simulink library "FoldingMechanisms"  (R2017a)
settings: Solver=VariableStepAuto  StartTime=0.0  StopTime=10.0  RelTol=1e-3
undefined symbols (not defined in the file or in its folder): X, Y, Z
libraries: sm_lib x70, FoldingMechanisms x62, nesl_utility x7
(part 4 of 4)

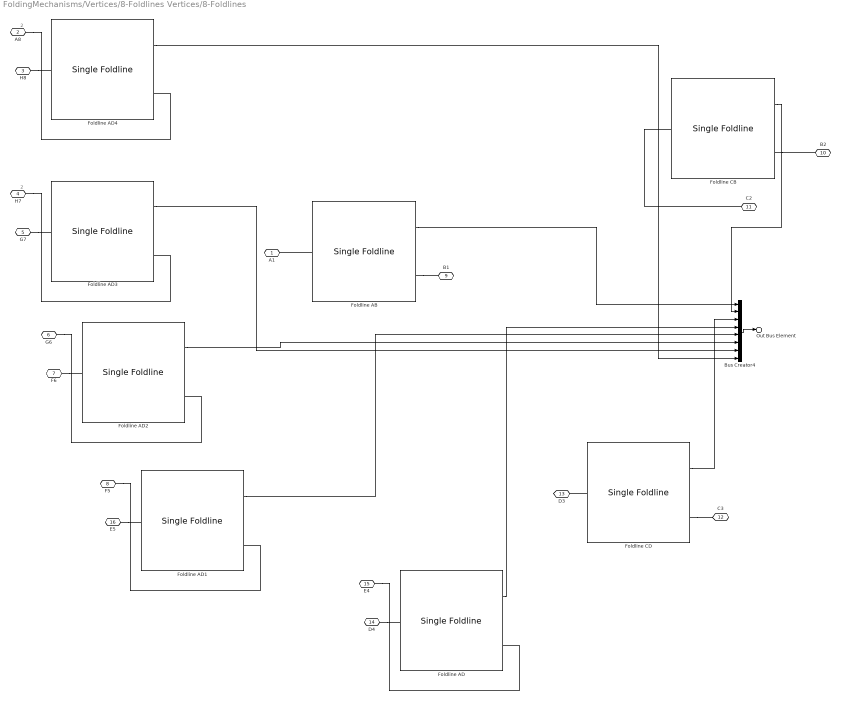
== system FoldingMechanisms/Vertices/8-Foldlines Vertices/8-Foldlines ==
  note: 2
  note: 2
  Bus Creator4 : BusCreator  Inputs=8
  Foldline AB : FoldingMechanisms/Vertices/Subelements/Single Foldline  angleAB=angval(1)  specAngleAB=angspec(1)
      settings: SourceProductName=FoldingMechanisms
  Foldline AD{,1..4} (5 alike) : FoldingMechanisms/Vertices/Subelements/Single Foldline  angleAB=angval(4)  specAngleAB=angspec(4)
      settings: SourceProductName=FoldingMechanisms
  Foldline CB : FoldingMechanisms/Vertices/Subelements/Single Foldline  angleAB=angval(2)  specAngleAB=angspec(2)
      settings: SourceProductName=FoldingMechanisms
  Foldline CD : FoldingMechanisms/Vertices/Subelements/Single Foldline  angleAB=angval(3)  specAngleAB=angspec(2)
      settings: SourceProductName=FoldingMechanisms
  A1 : PMIOPort  Port=1  Side=Left
  A8 : PMIOPort  Port=2  Side=Left
  H8 : PMIOPort  Port=3  Side=Left
  H7 : PMIOPort  Port=4  Side=Left
  G7 : PMIOPort  Port=5  Side=Left
  G6 : PMIOPort  Port=6  Side=Left
  F6 : PMIOPort  Port=7  Side=Left
  F5 : PMIOPort  Port=8  Side=Left
  B1 : PMIOPort  Port=9  Side=Right
  B2 : PMIOPort  Port=10  Side=Right
  C2 : PMIOPort  Port=11  Side=Right
  C3 : PMIOPort  Port=12  Side=Right
  D3 : PMIOPort  Port=13  Side=Right
  D4 : PMIOPort  Port=14  Side=Right
  E4 : PMIOPort  Port=15  Side=Right
  E5 : PMIOPort  Port=16  Side=Right
  Out Bus Element : Outport  PortName=OutBus  Element=Sensing
  wires:
  Foldline AD3/1 -> Bus Creator4/7
  Bus Creator4/1 -> Out Bus Element/1
  Foldline AB/1 -> Bus Creator4/1
  Foldline AD/1 -> Bus Creator4/4
  Foldline CD/1 -> Bus Creator4/3
  Foldline CB/1 -> Bus Creator4/2
  Foldline AD1/1 -> Bus Creator4/5
  Foldline AD2/1 -> Bus Creator4/6
  Foldline AD4/1 -> Bus Creator4/8
  connections:
  G7/RConn1 -- Foldline AD3/LConn1
  H7/RConn1 -- Foldline AD3/RConn1
  Foldline CB/RConn1 -- B2/RConn1
  Foldline AB/LConn1 -- A1/RConn1
  Foldline AB/RConn1 -- B1/RConn1
  D4/RConn1 -- Foldline AD/LConn1
  E4/RConn1 -- Foldline AD/RConn1
  Foldline CD/LConn1 -- D3/RConn1
  Foldline CD/RConn1 -- C3/RConn1
  C2/RConn1 -- Foldline CB/LConn1
  F5/RConn1 -- Foldline AD1/RConn1
  E5/RConn1 -- Foldline AD1/LConn1
  F6/RConn1 -- Foldline AD2/LConn1
  G6/RConn1 -- Foldline AD2/RConn1
  A8/RConn1 -- Foldline AD4/RConn1
  H8/RConn1 -- Foldline AD4/LConn1

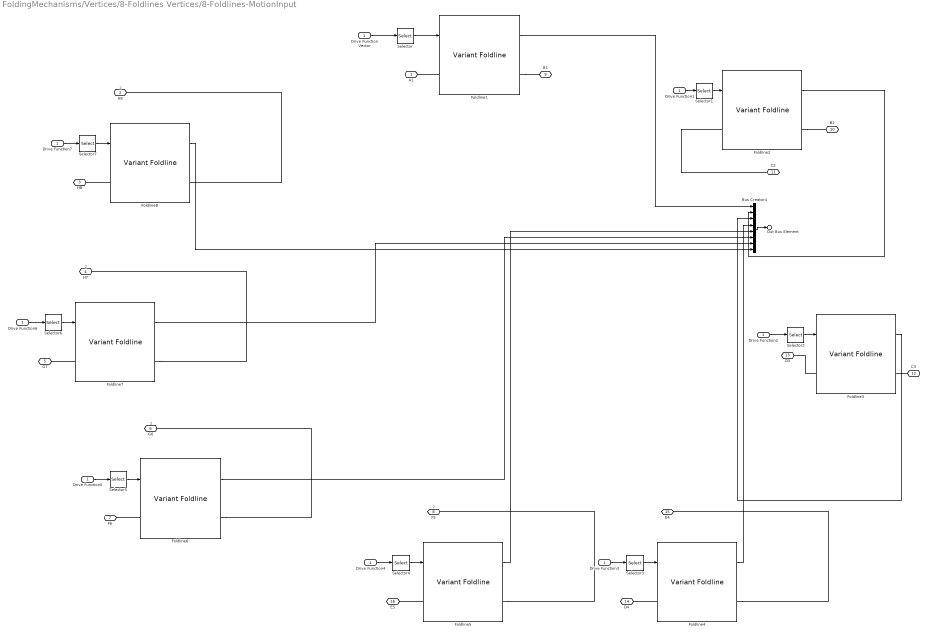
== system FoldingMechanisms/Vertices/8-Foldlines Vertices/8-Foldlines-MotionInput ==
  note: 2
  note: 2
  note: 2
  note: 2
  Drive Function Vector : Inport
  Bus Creator4 : BusCreator  Inputs=8
  Drive Function{1..7} (7 alike) : InportShadow
  Foldline1 : FoldingMechanisms/Vertices/Subelements/Variant Foldline  angleAB=angval(1)  specAngleAB=angspec(1)  actdrive=off  chooseVariant=Foldline
      settings: SourceProductName=FoldingMechanisms
  Foldline2 : FoldingMechanisms/Vertices/Subelements/Variant Foldline  angleAB=angval(2)  specAngleAB=angspec(2)  actdrive=off  chooseVariant=Foldline
      settings: SourceProductName=FoldingMechanisms
  Foldline3 : FoldingMechanisms/Vertices/Subelements/Variant Foldline  angleAB=angval(3)  specAngleAB=angspec(3)  actdrive=off  chooseVariant=Foldline
      settings: SourceProductName=FoldingMechanisms
  Foldline4 : FoldingMechanisms/Vertices/Subelements/Variant Foldline  angleAB=angval(4)  specAngleAB=angspec(4)  actdrive=off  chooseVariant=Foldline
      settings: SourceProductName=FoldingMechanisms
  Foldline5 : FoldingMechanisms/Vertices/Subelements/Variant Foldline  angleAB=angval(5)  specAngleAB=angspec(5)  actdrive=off  chooseVariant=Foldline
      settings: SourceProductName=FoldingMechanisms
  Foldline6 : FoldingMechanisms/Vertices/Subelements/Variant Foldline  angleAB=angval(6)  specAngleAB=angspec(6)  actdrive=off  chooseVariant=Foldline
      settings: SourceProductName=FoldingMechanisms
  Foldline7 : FoldingMechanisms/Vertices/Subelements/Variant Foldline  angleAB=angval(7)  specAngleAB=angspec(7)  actdrive=off  chooseVariant=Foldline
      settings: SourceProductName=FoldingMechanisms
  Foldline8 : FoldingMechanisms/Vertices/Subelements/Variant Foldline  angleAB=angval(7)  specAngleAB=angspec(7)  actdrive=off  chooseVariant=Foldline
      settings: SourceProductName=FoldingMechanisms
  Selector : Selector  InputPortWidth=max(n_actuation,1)  IndexOptions=Index vector (dialog)  Indices=inputselector(1)  OutputSizes=1
  Selector1 : Selector  InputPortWidth=max(n_actuation,1)  IndexOptions=Index vector (dialog)  Indices=inputselector(2)  OutputSizes=1
  Selector2 : Selector  InputPortWidth=max(n_actuation,1)  IndexOptions=Index vector (dialog)  Indices=inputselector(3)  OutputSizes=1
  Selector3 : Selector  InputPortWidth=max(n_actuation,1)  IndexOptions=Index vector (dialog)  Indices=inputselector(4)  OutputSizes=1
  Selector4 : Selector  InputPortWidth=max(n_actuation,1)  IndexOptions=Index vector (dialog)  Indices=inputselector(5)  OutputSizes=1
  Selector5 : Selector  InputPortWidth=max(n_actuation,1)  IndexOptions=Index vector (dialog)  Indices=inputselector(6)  OutputSizes=1
  Selector6 : Selector  InputPortWidth=max(n_actuation,1)  IndexOptions=Index vector (dialog)  Indices=inputselector(7)  OutputSizes=1
  Selector7 : Selector  InputPortWidth=max(n_actuation,1)  IndexOptions=Index vector (dialog)  Indices=inputselector(8)  OutputSizes=1
  A1 : PMIOPort  Port=1  Side=Left
  A8 : PMIOPort  Port=2  Side=Left
  H8 : PMIOPort  Port=3  Side=Left
  H7 : PMIOPort  Port=4  Side=Left
  G7 : PMIOPort  Port=5  Side=Left
  G6 : PMIOPort  Port=6  Side=Left
  F6 : PMIOPort  Port=7  Side=Left
  F5 : PMIOPort  Port=8  Side=Left
  B1 : PMIOPort  Port=9  Side=Right
  B2 : PMIOPort  Port=10  Side=Right
  C2 : PMIOPort  Port=11  Side=Right
  C3 : PMIOPort  Port=12  Side=Right
  D3 : PMIOPort  Port=13  Side=Right
  D4 : PMIOPort  Port=14  Side=Right
  E4 : PMIOPort  Port=15  Side=Right
  E5 : PMIOPort  Port=16  Side=Right
  Out Bus Element : Outport  PortName=OutBus  Element=Sensing
  wires:
  Foldline5/1 -> Bus Creator4/5
  Selector4/1 -> Foldline5/1
  Drive Function4/1 -> Selector4/1
  Selector3/1 -> Foldline4/1
  Selector2/1 -> Foldline3/1
  Selector1/1 -> Foldline2/1
  Selector/1 -> Foldline1/1
  Drive Function3/1 -> Selector3/1
  Drive Function2/1 -> Selector2/1
  Drive Function1/1 -> Selector1/1
  Foldline2/1 -> Bus Creator4/2
  Foldline3/1 -> Bus Creator4/3
  Foldline4/1 -> Bus Creator4/4
  Foldline1/1 -> Bus Creator4/1
  Drive Function Vector/1 -> Selector/1
  Bus Creator4/1 -> Out Bus Element/1
  Selector5/1 -> Foldline6/1
  Foldline6/1 -> Bus Creator4/6
  Drive Function5/1 -> Selector5/1
  Selector6/1 -> Foldline7/1
  Drive Function6/1 -> Selector6/1
  Foldline7/1 -> Bus Creator4/7
  Foldline8/1 -> Bus Creator4/8
  Drive Function7/1 -> Selector7/1
  Selector7/1 -> Foldline8/1
  connections:
  Foldline5/RConn1 -- F5/RConn1
  Foldline5/LConn1 -- E5/RConn1
  Foldline2/LConn1 -- C2/RConn1
  Foldline3/RConn1 -- C3/RConn1
  Foldline3/LConn1 -- D3/RConn1
  Foldline4/RConn1 -- E4/RConn1
  Foldline4/LConn1 -- D4/RConn1
  Foldline1/RConn1 -- B1/RConn1
  Foldline1/LConn1 -- A1/RConn1
  Foldline2/RConn1 -- B2/RConn1
  Foldline6/RConn1 -- G6/RConn1
  Foldline6/LConn1 -- F6/RConn1
  Foldline7/LConn1 -- G7/RConn1
  Foldline7/RConn1 -- H7/RConn1
  Foldline8/RConn1 -- A8/RConn1
  Foldline8/LConn1 -- H8/RConn1

== system FoldingMechanisms/Vertices/Subelements/Single Driven Foldline ==
  Drive Function : Inport
  Bus Creator : BusCreator  Inputs=3
  Foldline : sm_lib/Joints/Revolute Joint  SenseConstraintForce=off  SenseConstraintForceX=off  SenseConstraintForceY=off  SenseConstraintForceZ=off  SenseConstraintTorque=off  SenseConstraintTorqueX=off  SenseConstraintTorqueY=off  SenseConstraintTorqueZ=off  SenseTotalForce=off  SenseTotalForceX=off  SenseTotalForceY=off  SenseTotalForceZ=off  SenseTotalTorque=off  SenseTotalTorqueX=off  SenseTotalTorqueY=off  SenseTotalTorqueZ=off  CompositeWrenchDir=FollowerOnBase  CompositeWrenchFrame=BaseFrame  EquilibriumPosition=0  EquilibriumPositionUnits=deg  SpringStiffness=0  SpringStiffnessUnits=N*m/deg  DampingCoefficient=0  DampingCoefficientUnits=N*m/(deg/s)  TorqueActuationMode=ComputedTorque  MotionActuationMode=InputMotion  SensePosition=on  SenseVelocity=on  SenseAcceleration=off  SenseTorqueForce=on  PositionTargetSpecify=off  PositionTargetPriority=Low  PositionTargetValue=0  PositionTargetValueUnits=deg  VelocityTargetSpecify=off  VelocityTargetPriority=High  VelocityTargetValue=0  VelocityTargetValueUnits=deg/s
  PS-Simulink Converter : nesl_utility/PS-Simulink Converter  PhysicalDomain=network_engine_domain  SubClassName=ps_output  LeftPortType=input  RightPortType=output  PseudoPeriodic=off  Frequencies=[]  Unit=1  AffineConversion=off
  PS-Simulink Converter1 : nesl_utility/PS-Simulink Converter  PhysicalDomain=network_engine_domain  SubClassName=ps_output  LeftPortType=input  RightPortType=output  PseudoPeriodic=off  Frequencies=[]  Unit=1  AffineConversion=off
  PS-Simulink Converter2 : nesl_utility/PS-Simulink Converter  PhysicalDomain=network_engine_domain  SubClassName=ps_output  LeftPortType=input  RightPortType=output  PseudoPeriodic=off  Frequencies=[]  Unit=1  AffineConversion=off
  Simulink-PS Converter : nesl_utility/Simulink-PS Converter  PhysicalDomain=network_engine_domain  SubClassName=ps_input  LeftPortType=input  RightPortType=output  PseudoPeriodic=off  Frequencies=[]  NoiseDistribution=none  NoiseParameters=[]  Unit=1  AffineConversion=off  FilteringAndDerivatives=filter  SimscapeFilterOrder=2  InputFilterTimeConstant=0.001  UdotUserProvided=0
  Facet1 : PMIOPort  Port=1  Side=Left
  Facet2 : PMIOPort  Port=2  Side=Right
  Out Bus Element : Outport  PortName=OutBus  Element=Sensing
  wires:
  Drive Function/1 -> Simulink-PS Converter/1
  PS-Simulink Converter/1 -> Bus Creator/1  "s"
  PS-Simulink Converter1/1 -> Bus Creator/2  "v"
  PS-Simulink Converter2/1 -> Bus Creator/3  "T"
  Bus Creator/1 -> Out Bus Element/1  "AB"
  connections:
  Foldline/RConn1 -- Facet2/RConn1
  Foldline/LConn1 -- Facet1/RConn1
  Simulink-PS Converter/RConn1 -- Foldline/LConn2
  PS-Simulink Converter/LConn1 -- Foldline/RConn2
  PS-Simulink Converter1/LConn1 -- Foldline/RConn3
  PS-Simulink Converter2/LConn1 -- Foldline/RConn4

== system FoldingMechanisms/Vertices/Subelements/Single Foldline ==
  Bus Creator : BusCreator  Inputs=2
  Foldline : sm_lib/Joints/Revolute Joint  SenseConstraintForce=off  SenseConstraintForceX=off  SenseConstraintForceY=off  SenseConstraintForceZ=off  SenseConstraintTorque=off  SenseConstraintTorqueX=off  SenseConstraintTorqueY=off  SenseConstraintTorqueZ=off  SenseTotalForce=off  SenseTotalForceX=off  SenseTotalForceY=off  SenseTotalForceZ=off  SenseTotalTorque=off  SenseTotalTorqueX=off  SenseTotalTorqueY=off  SenseTotalTorqueZ=off  CompositeWrenchDir=FollowerOnBase  CompositeWrenchFrame=BaseFrame  EquilibriumPosition=0  EquilibriumPositionUnits=deg  SpringStiffness=0  SpringStiffnessUnits=N*m/deg  DampingCoefficient=0  DampingCoefficientUnits=N*m/(deg/s)  TorqueActuationMode=NoTorque  MotionActuationMode=ComputedMotion  SensePosition=on  SenseVelocity=on  SenseAcceleration=off  SenseTorqueForce=off  PositionTargetSpecify=off  PositionTargetPriority=Low  PositionTargetValue=angleAB  PositionTargetValueUnits=deg  VelocityTargetSpecify=off  VelocityTargetPriority=High  VelocityTargetValue=0  VelocityTargetValueUnits=deg/s
  PS-Simulink Converter : nesl_utility/PS-Simulink Converter  PhysicalDomain=network_engine_domain  SubClassName=ps_output  LeftPortType=input  RightPortType=output  PseudoPeriodic=off  Frequencies=[]  Unit=1  AffineConversion=off
  PS-Simulink Converter1 : nesl_utility/PS-Simulink Converter  PhysicalDomain=network_engine_domain  SubClassName=ps_output  LeftPortType=input  RightPortType=output  PseudoPeriodic=off  Frequencies=[]  Unit=1  AffineConversion=off
  Facet1 : PMIOPort  Port=1  Side=Left
  Facet2 : PMIOPort  Port=2  Side=Right
  Bus Element Out : Outport  PortName=OutBus  Element=Sensing
  wires:
  PS-Simulink Converter/1 -> Bus Creator/1  "s"
  PS-Simulink Converter1/1 -> Bus Creator/2  "v"
  Bus Creator/1 -> Bus Element Out/1
  connections:
  Foldline/LConn1 -- Facet1/RConn1
  Foldline/RConn1 -- Facet2/RConn1
  PS-Simulink Converter/LConn1 -- Foldline/RConn2
  PS-Simulink Converter1/LConn1 -- Foldline/RConn3

== system FoldingMechanisms/Vertices/Subelements/Variant Foldline ==
  note: 1) Add Subsystem or Model blocks as valid variant choices.
      | 2) You cannot connect blocks at this level. At simulation, connectivity is automatically
      | determined, based on the active variant and port name matching.
  DriveFunction : Inport
  Drive : Subsystem  VariantControl=Drive
  Foldline : Subsystem  VariantControl=Foldline
  Facet1 : PMIOPort  Port=1  Side=Left
  Facet2 : PMIOPort  Port=2  Side=Right
  OutBus : Outport

== system FoldingMechanisms/Vertices/Subelements/Variant Foldline/Drive ==
  DriveFunction : Inport
  Single Driven Foldline : FoldingMechanisms/Vertices/Subelements/Single Driven Foldline
      settings: SourceProductName=FoldingMechanisms
  Facet1 : PMIOPort  Port=1  Side=Left
  Facet2 : PMIOPort  Port=2  Side=Right
  OutBus : Outport
  wires:
  Single Driven Foldline/1 -> OutBus/1
  DriveFunction/1 -> Single Driven Foldline/1
  connections:
  Facet1/RConn1 -- Single Driven Foldline/LConn1
  Facet2/RConn1 -- Single Driven Foldline/RConn1

== system FoldingMechanisms/Vertices/Subelements/Variant Foldline/Foldline ==
  DriveFunction : Inport
  Single Foldline : FoldingMechanisms/Vertices/Subelements/Single Foldline  angleAB=angleAB  specAngleAB=specAngleAB
      settings: SourceProductName=FoldingMechanisms
  Terminator : Terminator
  Facet1 : PMIOPort  Port=1  Side=Left
  Facet2 : PMIOPort  Port=2  Side=Right
  OutBus : Outport
  wires:
  Single Foldline/1 -> OutBus/1
  DriveFunction/1 -> Terminator/1
  connections:
  Facet2/RConn1 -- Single Foldline/RConn1
  Facet1/RConn1 -- Single Foldline/LConn1
